simulink model "D3_test"  (R2019b)
settings: Solver=ode8  StartTime=0.0  StopTime=2  FixedStep=0.001000  RelTol=1e-3
settings Model: Creator=nahkusaidy  LastModifiedBy=nahkusaidy

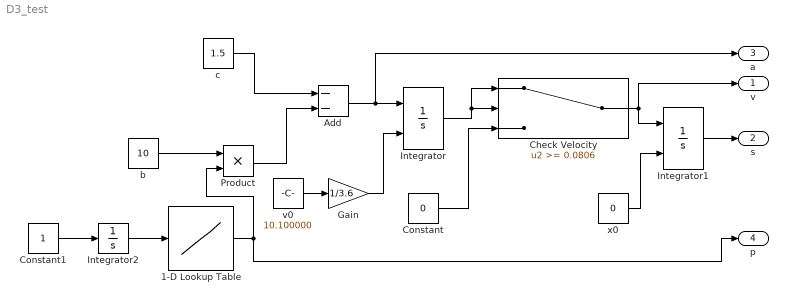
== system D3_test ==
  1-D Lookup Table : Lookup_n-D  NumberOfTableDimensions=1  BreakpointsForDimension1=[0 0.2 0.4 0.6 0.8 1 1.2]  Table=[0 .043 0.073 0.078 0.073 0.043 0.0]  ExtrapMethod=Clip  UseLastTableValue=on  InternalRulePriority=Speed  RndMeth=Simplest  InputSameDT=on
  Add : Sum  Inputs=--
  Check Velocity : Switch  Threshold=0.0806
  Constant : Constant  Value=0
  Constant1 : Constant
  Gain : Gain  Gain=1/3.6
  Integrator : Integrator  InitialConditionSource=external
  Integrator1 : Integrator  InitialConditionSource=external
  Integrator2 : Integrator
  Product : Product
  b : Constant  Value=10
  c : Constant  Value=1.5
  v0 : Constant  Value=10.100000
  x0 : Constant  Value=0
  v : Outport
  "s " : Outport  Port=2
  a : Outport  Port=3
  p : Outport  Port=4
  wires:
  c/1 -> Add/1
  b/1 -> Product/1
  Product/1 -> Add/2
  Add/1 -> a/1, Integrator/1
  Integrator/1 -> Check Velocity/1, Check Velocity/2
  Integrator1/1 -> "s "/1
  x0/1 -> Integrator1/2
  v0/1 -> Gain/1
  Gain/1 -> Integrator/2
  Constant/1 -> Check Velocity/3
  Check Velocity/1 -> Integrator1/1, v/1
  1-D Lookup Table/1 -> p/1, Product/2
  Constant1/1 -> Integrator2/1
  Integrator2/1 -> 1-D Lookup Table/1
